simulink model "mdl_GPSreceiveBin1_v3"  (R2020b)
settings: Solver=FixedStepAuto  StartTime=0.0  StopTime=10.0  FixedStep=0.01  RelTol=1e-3  EnableMultiTasking=on
libraries: simulink x3, raspberrypiCommlib x1
settings Model: Creator=cbeal  LastModifiedBy=cbeal
settings SolverCC: PositivePriorityOrder=on
settings DataIOCC: ReturnWorkspaceOutputs=off
settings OptimizationCC: EnhancedBackFolding=on  PassReuseOutputArgsAs=Individual arguments  ZeroExternalMemoryAtStartup=off  ZeroInternalMemoryAtStartup=off  MaxStackSize=64  OptimizeBlockOrder=speed  DifferentSizesBufferReuse=on  OptimizationCustomize=off  EfficientTunableParamExpr=on
settings DebuggingCC: ParameterTunabilityLossMsg=error
settings HardwareCC: ProdBitPerPointer=32  ProdBitPerSizeT=32  ProdBitPerPtrDiffT=32  ProdLargestAtomicInteger=Long  ProdLargestAtomicFloat=Double  ProdWordSize=32  ProdLongLongMode=on  ProdHWDeviceType=ARM Compatible->ARM Cortex
settings RTWCC: Description=Embedded Coder  SystemTargetFile=ert.tlc  HardwareBoard=Raspberry Pi  TLCOptions="-aInlineSetEventsForThisBaseRateFcn=TLC_FALSE -aSuppressMultiTaskScheduler=TLC_FALSE  -aRateBasedStepFcn=0"  TemplateMakefile=ert_default_tmf  Toolchain=GNU GCC Raspberry Pi  BuildConfiguration=Faster Runs
settings CodeAppCC: ForceParamTrailComments=on  IgnoreCustomStorageClasses=off  OperatorAnnotations=on  SimulinkDataObjDesc=on  SFDataObjDesc=on  InsertBlockDesc=on
settings ERTTargetCC: MatFileLogging=on  SupportVariableSizeSignals=on  ExtModeTransport=2  ExtModeMexFile=ext_xcp  ExtModeIntrfLevel=Level2 - Open

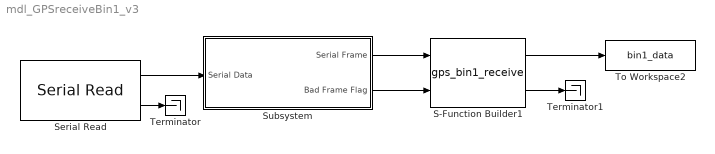
== system mdl_GPSreceiveBin1_v3 ==
  S-Function Builder1 : S-Function  FunctionName=gps_bin1_receive  SFunctionModules=gps_bin1_receive_wrapper  SFunctionDeploymentMode=off  EnableBusSupport=off  mask(S-Function Builder){}
      mask help: Simulink:masks:SFunctionBuilder_MD
      mask init:
      | val = [[.9  0.75 0.75 1 1 .9 .9 1]',[1 1 0.75 0.75 .9 .9 1 .9]'];try , sys = get_param(gcb,'SfunBuilderFcnName');if isempty(sys), sys = get_param(gcb,'FunctionName'); end,catch, sys = get_param(gcb,'FunctionName'); end
      settings: CopyFcn=set_param(gcbh,'LinkStatus','none')  OpenFcn=sfunctionwizard(gcbh)
      mask Display:
      | plot(val(:,1),val(:,2))
      | disp(sys)
      | port_label('input',1,'u0')
      | port_label('input',2,'u1')
      | port_label('output',1,'y0')
      | port_label('output',2,'y1')
  Serial Read : raspberrypiCommlib/Serial Read  board=Pi 3 Model B  SCIModule_=/dev/serial0  Baudrate_=19200  Parity=None  StopBits_=1  HardwareFlowControl=None  ByteOrder=LittleEndian  DataLength=64  DataType=uint8  OutputStatus=on  SampleTime=-1  blockPlatform=RaspberryPi
      settings: SourceProductBaseCode=RASPPI
  Subsystem : Subsystem
  Terminator : Terminator
  Terminator1 : Terminator
  To Workspace2 : ToWorkspace  VariableName=bin1_data  SampleTime=-1
      settings: Save2DSignal=2-D array (concatenate along first dimension)
  wires:
  Subsystem/1(Serial Frame) -> S-Function Builder1/1
  Subsystem/2(Bad Frame Flag) -> S-Function Builder1/2
  S-Function Builder1/2 -> Terminator1/1
  Serial Read/1 -> Subsystem/1(Serial Data)
  Serial Read/2 -> Terminator/1
  S-Function Builder1/1 -> To Workspace2/1

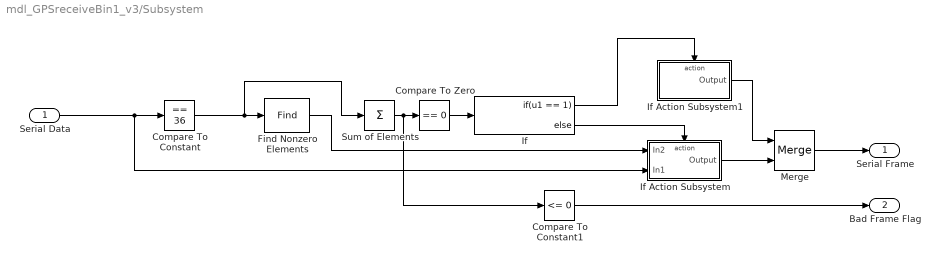
== system mdl_GPSreceiveBin1_v3/Subsystem ==
  Serial Data : Inport
  Compare To Constant : simulink/Logic and Bit Operations/Compare To Constant  relop===  const=36  OutDataTypeStr=boolean
  Compare To Constant1 : simulink/Logic and Bit Operations/Compare To Constant  relop=<=  const=0  OutDataTypeStr=uint8
  Compare To Zero : simulink/Logic and Bit Operations/Compare To Zero  relop===  OutDataTypeStr=boolean
  Find Nonzero Elements : Find  NumberOfInputDimensions=3
  If : If  IfExpression=u1 == 1
  If Action Subsystem : Subsystem  TreatAsAtomicUnit=on
  If Action Subsystem1 : Subsystem  TreatAsAtomicUnit=on
  Merge : Merge
  Sum of Elements : Sum  Inputs=+
  Serial Frame : Outport
  Bad Frame Flag : Outport  Port=2
  wires:
  Compare To Constant1/1 -> Bad Frame Flag/1
  Find Nonzero Elements/1 -> If Action Subsystem/1(In2)
  Sum of Elements/1 -> Compare To Constant1/1, Compare To Zero/1
  If Action Subsystem1/1(Output) -> Merge/1
  Compare To Constant/1 -> Sum of Elements/1, Find Nonzero Elements/1
  Compare To Zero/1 -> If/1
  If/1 -> If Action Subsystem1/Action
  If/2 -> If Action Subsystem/Action
  If Action Subsystem/1(Output) -> Merge/2
  Serial Data/1 -> If Action Subsystem/2(In1), Compare To Constant/1
  Merge/1 -> Serial Frame/1

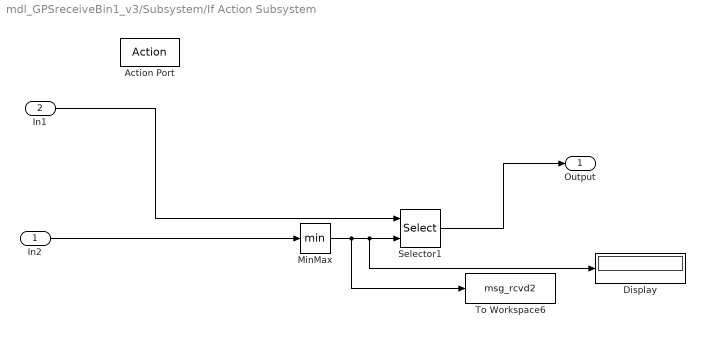
== system mdl_GPSreceiveBin1_v3/Subsystem/If Action Subsystem ==
  In2 : Inport
  In1 : Inport  Port=2
  Action Port : ActionPort  ActionPortLabel=else
  Display : Display
  MinMax : MinMax
  Selector1 : Selector  InputPortWidth=64  IndexOptions=Starting index (port)  Indices=[1 3]  OutputSizes=64
  To Workspace6 : ToWorkspace  VariableName=msg_rcvd2  SampleTime=-1
      settings: Save2DSignal=2-D array (concatenate along first dimension)
  Output : Outport
  wires:
  Selector1/1 -> Output/1
  In1/1 -> Selector1/1
  MinMax/1 -> Selector1/2, Display/1, To Workspace6/1
  In2/1 -> MinMax/1

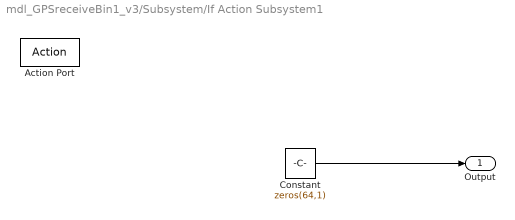
== system mdl_GPSreceiveBin1_v3/Subsystem/If Action Subsystem1 ==
  Action Port : ActionPort  ActionPortLabel=if(u1 == 1)
  Constant : Constant  Value=zeros(64,1)  OutDataTypeStr=uint8
  Output : Outport
  wires:
  Constant/1 -> Output/1
